simulink model "s0508_IVC_OpenLoop"  (R2021a)
settings: Solver=FixedStepAuto  StartTime=0.0  StopTime=10.0  FixedStep=0.001  RelTol=1e-3
libraries: CarMaker4SL x4
settings Model: Creator=jason  LastModifiedBy=jason

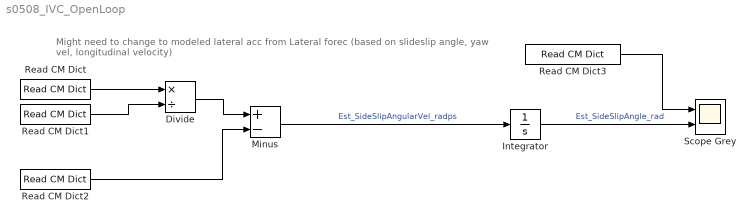
== system s0508_IVC_OpenLoop ==
  note: Might need to change to modeled lateral acc from Lateral forec (based on slideslip angle, yaw vel, longitudinal velocity)
  Divide : Product  Inputs=*/
  Integrator : Integrator
  Minus : Sum  Inputs=+-
  Read CM Dict : CarMaker4SL/Read CM Dict  xname=Car.ay  xsync=off  xstime=Continuous
  Read CM Dict1 : CarMaker4SL/Read CM Dict  xname=Car.vx  xsync=off  xstime=Continuous
  Read CM Dict2 : CarMaker4SL/Read CM Dict  xname=Car.YawVel  xsync=off  xstime=Continuous
  Read CM Dict3 : CarMaker4SL/Read CM Dict  xname=Car.SideSlipAngle  xsync=off  xstime=Continuous
  Scope Grey : Scope  NumInputPorts=2
  wires:
  Integrator/1 -> Scope Grey/2  "Est_SideSlipAngle_rad"
  Minus/1 -> Integrator/1  "Est_SideSlipAngularVel_radps"
  Read CM Dict/1 -> Divide/1
  Read CM Dict1/1 -> Divide/2
  Divide/1 -> Minus/1
  Read CM Dict2/1 -> Minus/2
  Read CM Dict3/1 -> Scope Grey/1
